simulink model "HVDC_MMC1_EMT"  (R2023b)
settings: Solver=ode23tb  StartTime=0.0  StopTime=10  MaxStep=Ts  RelTol=1e-3  EnableMultiTasking=on
PreLoadFcn:
  | HVDC_MMC_param
StartFcn:
  | tic
StopFcn:
  | toc
values from neighbouring files (symbols this model uses):
  acdcV = 1/(Vnom_dc/2*sqrt(3)/sqrt(2)/Vnom_sec)    [HVDC_MMC_param.m]
  C_PM = 1.758e-3    (= 0.001758)    [HVDC_MMC_param.m]
  Carm = 1.0*C_pm/n    (= 0.0002096)    [B2B_HVDC_MMC_Calc.m]    (also in HVDC_MMC_param.m = 4.88333333333e-05)
  DC_cable_C_shunt = 0.1e-6    (= 1e-07)    [HVDC_MMC_param.m]
  DC_cable_R_shunt = 1000    [HVDC_MMC_param.m]
  DCM = 1    [HVDC_MMC_param.m]
  Fn_filter = 1000    [B2B_HVDC_MMC_Calc.m]    (also in HVDC_MMC_param.m)
  Fnom = 50    [HVDC_MMC_param.m]
  HRM = 2    [HVDC_MMC_param.m]
  HrmOrd = N    (= 2)    [B2B_HVDC_MMC_Calc.m]    (also in HVDC_MMC_param.m)
  Ib_ac = (2/3)*Pnom/Vb_ac    [HVDC_MMC_param.m]
  Ib_dc = Pnom/Vb_dc    (= 1501.5015015)    [HVDC_MMC_param.m]
  Ki_CCSC = 50    [HVDC_MMC_param.m]
  Ki_Ireg = 6    [HVDC_MMC_param.m]
  Ki_Preg = 1.0    (= 1)    [HVDC_MMC_param.m]
  Ki_Qreg = 1.0    (= 1)    [HVDC_MMC_param.m]
  Ki_VDCreg = 100    [HVDC_MMC_param.m]
  Kp_CCSC = 0.8    [HVDC_MMC_param.m]
  Kp_Ireg = 0.6    [HVDC_MMC_param.m]
  Kp_Preg = 0.5/3    (= 0.166666666667)    [HVDC_MMC_param.m]
  Kp_Qreg = 0.5/3    (= 0.166666666667)    [HVDC_MMC_param.m]
  Kp_VDCreg = 4    [HVDC_MMC_param.m]
  L_cable = 15e-3    (= 0.015)    [HVDC_MMC_param.m]
  Larm = Larm_pu*(Zb_ac/w)    [HVDC_MMC_param.m]
  Lff = Larm_pu/2+Lxfo    (= 0.195)    [HVDC_MMC_param.m]
  Limits_Ireg = [ 2.0  -2.0]    [HVDC_MMC_param.m]
  Limits_Preg = [ 1.2, 0.8 ]    [HVDC_MMC_param.m]
  Limits_Qreg = [ 0.25, -0.25 ]    [HVDC_MMC_param.m]
  Limits_VDCreg = [ 2.0  -2.0]    [HVDC_MMC_param.m]
  Lxfo = 0.12    [HVDC_MMC_param.m]
  Pac = 0.9    [HVDC_MMC_param.m]
  Pnom = 1000e6    (= 1000000000)    [HVDC_MMC_param.m]
  Qac = 0.2    [HVDC_MMC_param.m]
  QCM = 0    [HVDC_MMC_param.m]
  R_cable = 0.5    [HVDC_MMC_param.m]
  Rarm = Rarm_pu*Zb_ac    [HVDC_MMC_param.m]
  Rff = Rarm_pu/2+Rxfo    (= 0.00375)    [HVDC_MMC_param.m]
  Rxfo = 0.003    [HVDC_MMC_param.m]
  Slope_Pref = 0.5    [HVDC_MMC_param.m]
  Slope_Qref = 0.5    [HVDC_MMC_param.m]
  Slope_Vdc_ref = Vnom_dc/5    (= 133200)    [HVDC_MMC_param.m]
  Tbrk1_On = 0.1    [HVDC_MMC_param.m]
  Tbrk2_On = 1.0    (= 1)    [HVDC_MMC_param.m]
  Tdeblock = 1.5    [HVDC_MMC_param.m]
  Tfault = 9999    [HVDC_MMC_param.m]
  Ton_Converter2 = 3    [HVDC_MMC_param.m]
  Ton_PQreg = 2    [HVDC_MMC_param.m]
  Ton_VDCreg = 1.5    [HVDC_MMC_param.m]
  Ts = Ts_Power    (= 5e-05)    [B2B_HVDC_MMC_Calc.m]    (also in HVDC_MMC_param.m)
  Ts_Control = Ts_Power    (= 5e-05)    [B2B_HVDC_MMC_Calc.m]    (also in HVDC_MMC_param.m)
  Ts_DQN = MultTs*Ts_Power    (= 5e-05)    [B2B_HVDC_MMC_Calc.m]    (also in HVDC_MMC_param.m)
  Ts_EMT = Ts    (= 5e-05)    [HVDC_MMC_param.m]
  Ts_Power = 1*50e-6    (= 5e-05)    [B2B_HVDC_MMC_Calc.m]    (also in HVDC_MMC_param.m)
  Vb_ac = sqrt(2/3)*Vnom_sec    [HVDC_MMC_param.m]
  Vb_dc = Vnom_dc    (= 666000)    [HVDC_MMC_param.m]
  Vc0_PM = 0    [HVDC_MMC_param.m]
  Vnom_dc = 2*Vnom_sec    (= 666000)    [HVDC_MMC_param.m]
  Vnom_prim = 333e3    (= 333000)    [HVDC_MMC_param.m]
  Vnom_sec = 333e3    (= 333000)    [HVDC_MMC_param.m]
  w = 2*pi*f    (= 314.159265359)    [B2B_HVDC_MMC_Calc.m]    (also in HVDC_MMC_param.m)
  Ws = 2*pi*Fnom    (= 314.159265359)    [HVDC_MMC_param.m]
  Zb_ac = Vb_ac/Ib_ac    [HVDC_MMC_param.m]
  Zeta_filter = 1    [B2B_HVDC_MMC_Calc.m]    (also in HVDC_MMC_param.m)
undefined symbols (not defined in the file or in its folder): DCss, DiscIntNeverNeededParam, gcbh, MT, sps_rtmsupport
libraries: DQN_Lib x37, simulink x35, spsCurrentMeasurementLib x24, powerlib_extras x21, slpidlib x14, spsSecondOrderFilterLib x14, spsVoltageMeasurementLib x10, spsSeriesRLCBranchLib x10, spsControlledVoltageSourceLib x9, spsHalfBridgeMMCmodel x7, spsGroundLib x4, spsParallelRLCBranchLib x4
(part 9 of 9)

== matlab function HVDC_MMC1_EMT/MMC_DQN/MATLAB Function2 ==
  data: Ydcpnz_c output; X_DQN input
function Ydcpnz_c  = fDQN012C(X_DQN)
        
            if(size(X_DQN,2) < 1)
                error('Wrong size!');
            end
            
            N = size(X_DQN,1);
        
            if(size(X_DQN,1) == 6 && size(X_DQN,2) == 1)
                N = 1;
                X_DQN = X_DQN';
            end
        
            Ydcpnz_c = complex(zeros(3,N));
        
            for i = 1 : N
             
                if(i>1)
                    Ydcpnz_c(1,i) = (X_DQN(i,1)) + 1i*X_DQN(i,4);
                    Ydcpnz_c(2,i) = (-X_DQN(i,2)) + 1i*X_DQN(i,5);
                    Ydcpnz_c(3,i) = (X_DQN(i,3)) + 1i*X_DQN(i,6);
                else
        
                    Ydcpnz_c(1,i) = 0.5*(X_DQN(i,4) - 1i*X_DQN(i,1));
                    Ydcpnz_c(2,i) = 0.5*(X_DQN(i,5) + 1i*X_DQN(i,2));
                    Ydcpnz_c(3,i) =     (X_DQN(i,6) + 1i*X_DQN(i,3));
                end
            
            end
        
        
end

== matlab function HVDC_MMC1_EMT/MMC_ABC/MATLAB Function1 ==
  data: m1_dq input; m2_dq input; mp_c output; N parameter; mn_c output
function [mp_c, mn_c]   = fDQN012c(m1_dq, m2_dq, N)


    mp_c  = complex(zeros(3, N+1));
    mn_c  = complex(zeros(3, N+1));
    % Vr1_c = complex(zeros(3, N+1));
    % Vr2_c = complex(zeros(3, N+1));


    mp_c(3,1)  = 0.5;
    mp_c(1,2)  = -0.5*(m1_dq(1) + 1i*m1_dq(2));
    mp_c(2,3)  = -0.5*(m2_dq(1) - 1i*m2_dq(2));

    mn_c(3,1)  = 0.5;
    mn_c(1,2)  = 0.5*(m1_dq(1) + 1i*m1_dq(2));
    mn_c(2,3)  = -0.5*(m2_dq(1) - 1i*m2_dq(2));



    %mp_c(2,3)  = -m2_dq(1) - 1i*m2_dq(2);
    % Vr1_c(1,2) = Vdq_vec(3) + 1i*Vdq_vec(4);
    % Vr2_c(1,2) = Vdq_vec(5) + 1i*Vdq_vec(6);



end

== matlab function HVDC_MMC1_EMT/MMC/Half-Bridge MMC Ap/Model/MATLAB Function2 ==
  data: g input; V output; Vdc input; n parameter; ModelType parameter
function V  = FunctionDiscrete1(g, Vdc, n, ModelType)
[V]=FunctionHalfBridgeMMC1(g,Vdc, n, ModelType);

== matlab function HVDC_MMC1_EMT/MMC_DQN/MATLAB Function3 ==
  data: Vdq_vec input; Vs_c output; N parameter
function Vs_c   = fDQN012c(Vdq_vec, N)


    Vs_c  = complex(zeros(3, N+1));
    % Vr1_c = complex(zeros(3, N+1));
    % Vr2_c = complex(zeros(3, N+1));

    Vs_c(1,2)  = Vdq_vec(1) + 1i*Vdq_vec(2);
    % Vr1_c(1,2) = Vdq_vec(3) + 1i*Vdq_vec(4);
    % Vr2_c(1,2) = Vdq_vec(5) + 1i*Vdq_vec(6);



end

== matlab function HVDC_MMC1_EMT/MMC_DQN/MATLAB Function5 ==
  data: Vdq_vec input; Vs_c output; N parameter
function Vs_c   = fDQN012c(Vdq_vec, N)


    Vs_c  = complex(zeros(3, N+1));
    % Vr1_c = complex(zeros(3, N+1));
    % Vr2_c = complex(zeros(3, N+1));

    Vs_c(1,2)  = Vdq_vec(1) + 1i*Vdq_vec(2);
    % Vr1_c(1,2) = Vdq_vec(3) + 1i*Vdq_vec(4);
    % Vr2_c(1,2) = Vdq_vec(5) + 1i*Vdq_vec(6);



end

== matlab function HVDC_MMC1_EMT/MMC_ABC/MATLAB Function2 ==
  data: Vdc input; Vdc_c output; N parameter
function Vdc_c    = Vdc2c(Vdc, N)


    Vdc_c  = complex(zeros(3, N+1));

    Vdc_c(3,1)  = Vdc;



end
